simulink model "untitled"  (R2018b)
settings: Solver=VariableStepAuto  StartTime=0.0  StopTime=10.0  RelTol=1e-3
settings Model: Creator=jhoysbou  LastModifiedBy=jhoysbou

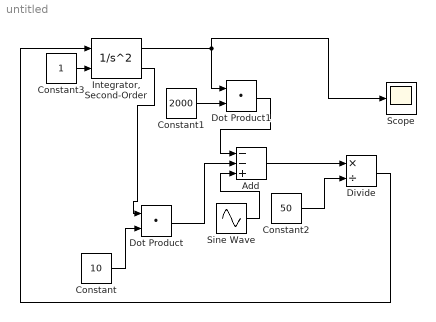
== system untitled ==
  Add : Sum  Inputs=--+
  Constant : Constant  Value=10
  Constant1 : Constant  Value=2000
  Constant2 : Constant  Value=50
  Constant3 : Constant
  Divide : Product  Inputs=*/
  Dot Product : DotProduct  InputSameDT=on  OutDataTypeStr=Inherit: Inherit via internal rule
  Dot Product1 : DotProduct  InputSameDT=on  OutDataTypeStr=Inherit: Inherit via internal rule
  "Integrator, Second-Order" : SecondOrderIntegrator  ICSourceX=external
  Scope : Scope
  Sine Wave : Sin  Amplitude=10  SampleTime=0
  wires:
  Constant/1 -> Dot Product/2
  Dot Product/1 -> Add/2
  Sine Wave/1 -> Add/3
  "Integrator, Second-Order"/1 -> Scope/1, Dot Product1/1
  Constant1/1 -> Dot Product1/2
  Dot Product1/1 -> Add/1
  Add/1 -> Divide/1
  Constant2/1 -> Divide/2
  Divide/1 -> "Integrator, Second-Order"/1
  "Integrator, Second-Order"/2 -> Dot Product/1
  Constant3/1 -> "Integrator, Second-Order"/2
